simulink model "test"  (R2018a)
settings: Solver=VariableStepAuto  StartTime=0.0  StopTime=10.0  RelTol=1e-3
settings Model: Creator=jonathan  LastModifiedBy=jonathan

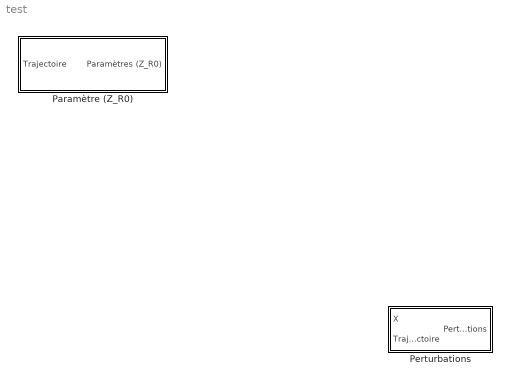
== system test ==
  Paramètre (Z_R0) : Subsystem
  Perturbations : Subsystem

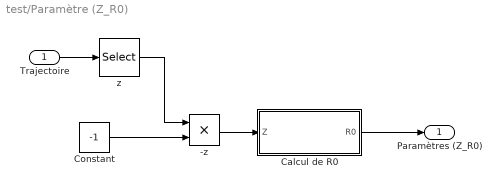
== system test/Paramètre (Z_R0) ==
  Trajectoire : Inport
  -z : Product
  Calcul de R0 : Subsystem
  Constant : Constant  Value=-1
  z : Selector  InputPortWidth=3  IndexOptions=Index vector (dialog)  Indices=3  OutputSizes=1
  Paramètres (Z_R0) : Outport
  wires:
  Trajectoire/1 -> z/1
  Constant/1 -> -z/2
  z/1 -> -z/1
  -z/1 -> Calcul de R0/1(Z)
  Calcul de R0/1(R0) -> Paramètres (Z_R0)/1

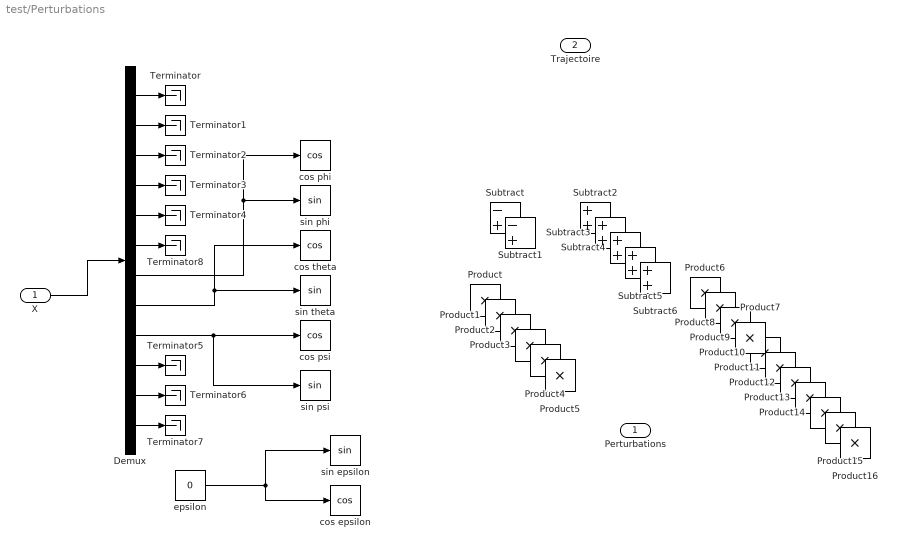
== system test/Perturbations ==
  X : Inport
  Trajectoire : Inport  Port=2
  Demux : Demux  Outputs=12
  Product{,1..5} (6 alike) : Product  Inputs=3
  Product{6..16} (11 alike) : Product
  Subtract : Sum  Inputs=-+
  Subtract1 : Sum  Inputs=-+
  Subtract{2..6} (5 alike) : Sum
  Terminator{,1..8} (9 alike) : Terminator
  cos epsilon : Trigonometry  Operator=cos
  cos phi : Trigonometry  Operator=cos
  cos psi : Trigonometry  Operator=cos
  cos theta : Trigonometry  Operator=cos
  epsilon : Constant  Value=0
  sin epsilon : Trigonometry
  sin phi : Trigonometry
  sin psi : Trigonometry
  sin theta : Trigonometry
  Perturbations : Outport
  wires:
  Demux/1 -> Terminator/1
  Demux/2 -> Terminator1/1
  Demux/3 -> Terminator2/1
  Demux/4 -> Terminator3/1
  Demux/5 -> Terminator4/1
  Demux/10 -> Terminator5/1
  Demux/11 -> Terminator6/1
  Demux/12 -> Terminator7/1
  Demux/6 -> Terminator8/1
  X/1 -> Demux/1
  Demux/7 -> sin phi/1, cos phi/1
  Demux/8 -> sin theta/1, cos theta/1
  Demux/9 -> cos psi/1, sin psi/1
  epsilon/1 -> cos epsilon/1, sin epsilon/1

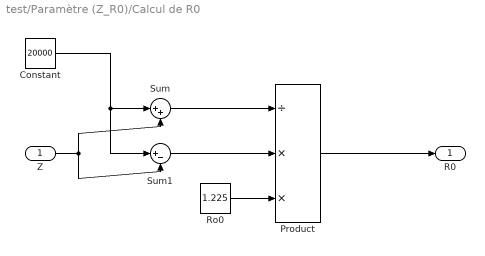
== system test/Paramètre (Z_R0)/Calcul de R0 ==
  Z : Inport
  Constant : Constant  Value=20000
  Product : Product  Inputs=/**
  Ro0 : Constant  Value=1.225
  Sum : Sum  Inputs=|++
  Sum1 : Sum  Inputs=|+-
  R0 : Outport
  wires:
  Constant/1 -> Sum1/1, Sum/1
  Z/1 -> Sum1/2, Sum/2
  Product/1 -> R0/1
  Sum1/1 -> Product/2
  Sum/1 -> Product/1
  Ro0/1 -> Product/3
